simulink library "jets_control_v1"  (R2021b)
settings: Solver=VariableStepAuto  StartTime=0.0  StopTime=10.0  RelTol=1e-3
undefined symbols (not defined in the file): Config, DiscIntNeverNeededParam
settings Model: Creator=gnava  LastModifiedBy=gnava
settings SolverCC: AlgebraicLoopSolver=TrustRegion
settings DebuggingCC: SFMachineParentedDataDiag=warning

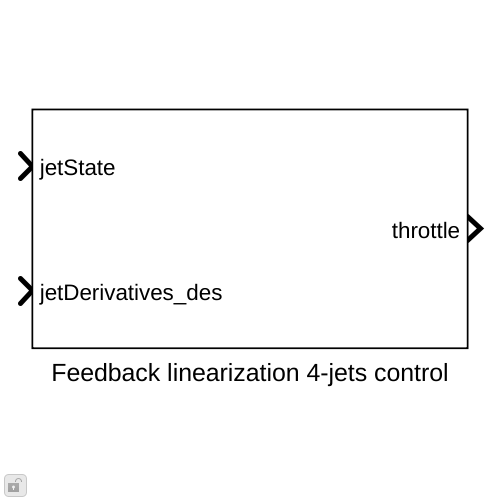
[thumbnail: Simulink's stored preview of the top-level diagram]
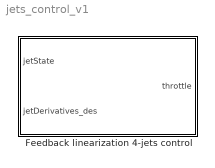
== system jets_control_v1 ==
  Feedback linearization 4-jets control : Subsystem  mask{Conf=Config}
      mask prompts: Conf "Configuration structure"
      mask DialogControl DescTextVar Prompt: Feedback linearization based controller for the 4 jets. This block takes as input the state (thrust and its rate-of-change) of the 4 jets and the desired rate-of-change of the thrust. The full state usually comes from an observer (e.g. an EKF). The output of this block is the throttle for the 4 jets.

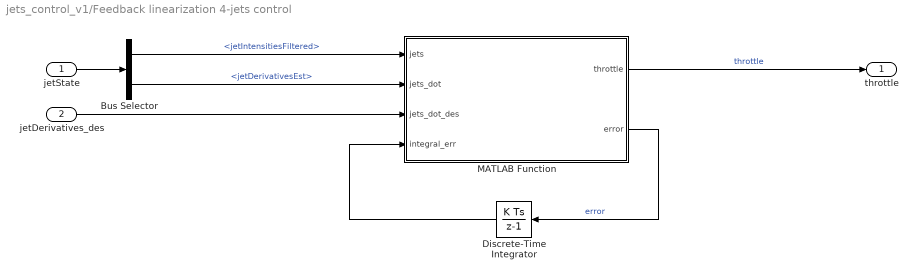
== system jets_control_v1/Feedback linearization 4-jets control ==
  jetState : Inport
  jetDerivatives_des : Inport  Port=2
  Bus Selector : BusSelector  OutputSignals=jetIntensitiesFiltered,jetDerivativesEst
  Discrete-Time Integrator : DiscreteIntegrator  SampleTime=Config.tStep  ICPrevOutput=DiscIntNeverNeededParam  ICPrevScaledInput=DiscIntNeverNeededParam
  MATLAB Function : MATLAB Function  TreatAsAtomicUnit=on
  throttle : Outport  VectorParamsAs1DForOutWhenUnconnected=off
  wires:
  Bus Selector/1 -> MATLAB Function/1(jets)  "<jetIntensitiesFiltered>"
  MATLAB Function/1(throttle) -> throttle/1  "throttle"
  jetState/1 -> Bus Selector/1
  MATLAB Function/2(error) -> Discrete-Time Integrator/1  "error"
  Bus Selector/2 -> MATLAB Function/2(jets_dot)  "<jetDerivativesEst>"
  Discrete-Time Integrator/1 -> MATLAB Function/4(integral_err)
  jetDerivatives_des/1 -> MATLAB Function/3(jets_dot_des)

== matlab function jets_control_v1/Feedback linearization 4-jets control/MATLAB Function ==
  data: jets input; jets_dot input; jets_dot_des input; throttle output size=[4,1]; Config parameter; error output; integral_err input
function [throttle, error]  = fl_jets_control(jets, jets_dot, jets_dot_des, Config, integral_err)

[throttle, error]  = iRonCubLib_v1.fl_jets_control(jets, jets_dot, jets_dot_des, Config, integral_err);
end
